simulink model "FinalSim"  (R2022b)
settings: Solver=VariableStepAuto  StartTime=0.0  StopTime=10  RelTol=1e-3
libraries: eeGeneralControl x3
(part 7 of 7)

== system FinalSim/Shoulder Transverse Model/Shoulder Transverse Flexors1/fascicles (CE & PE)/Type F Motor Units/Motor Unit 3 ==
  fenv : Inport
  Y,L : Inport  Port=2
  1/Tf (feff' < 0) : Fcn  Expr=u(2)/(0.02822+0.01513*u(3))
  1/Tf (feff' > 0) : Fcn  Expr=1/(0.02057*u(2)^2+0.0136*u(4))
  1/Ts : Gain  Gain=23.2558  SaturateOnIntegerOverflow=on  OutDataTypeStr=Inherit: Same as input  ParamDataTypeStr=Inherit: Same as input
  Af : Fcn  Expr=1-exp(-(u(1)*u(4)*u(3)/(0.56*u(2)))^u(2))
  Leff' : Fcn  Expr=(u(2)-u(1))^3/((1-u(3))*8.8e-005)
  Leff'->Leff : Integrator  InitialCondition=1
  "Leff,L, Af,fenv" : Mux
  S and old S diff : Sum  Inputs=-+  InputSameDT=on  SaturateOnIntegerOverflow=on  OutDataTypeStr=Inherit: Same as first input
  Y,nf,feff,S : Mux
  aS1 : Constant  Value=1.76
  aS2 : Constant  Value=0.96
  demux Y,L : Demux  Outputs=2
      settings: DisplayOption=none
  feff' : Product  InputSameDT=on  RndMeth=Zero  SaturateOnIntegerOverflow=on  OutDataTypeStr=Inherit: Same as first input
  feff' > 0? : Switch
  feff'->feff : Integrator
  feff>0.1? : Switch  Threshold=0.1
  fenv-fint : Sum  Inputs=+-  InputSameDT=on  SaturateOnIntegerOverflow=on  OutDataTypeStr=Inherit: Same as first input
  fint' : Product  InputSameDT=on  RndMeth=Zero  SaturateOnIntegerOverflow=on  OutDataTypeStr=Inherit: Same as first input
  fint'->fint : Integrator
  fint-feff : Sum  Inputs=+-  InputSameDT=on  SaturateOnIntegerOverflow=on  OutDataTypeStr=Inherit: Same as first input
  nf : Fcn  Expr=2.11+3.31*(1/u-1)
  s'->s : Integrator  InitialCondition=1.76
  A : Outport
  wires:
  Y,L/1 -> demux Y,L/1
  demux Y,L/1 -> Y,nf,feff,S/1
  demux Y,L/2 -> "Leff,L, Af,fenv"/2
  "Leff,L, Af,fenv"/1 -> 1/Tf (feff' < 0)/1, Leff'/1, 1/Tf (feff' > 0)/1
  1/Tf (feff' > 0)/1 -> feff' > 0?/1
  1/Tf (feff' < 0)/1 -> feff' > 0?/3
  fenv/1 -> fenv-fint/1, "Leff,L, Af,fenv"/4
  fenv-fint/1 -> fint'/2
  fint'/1 -> fint'->fint/1
  fint'->fint/1 -> fint-feff/1, fenv-fint/2
  fint-feff/1 -> feff'/2, feff' > 0?/2
  feff' > 0?/1 -> feff'/1, fint'/1
  feff'/1 -> feff'->feff/1
  feff'->feff/1 -> fint-feff/2, Y,nf,feff,S/3, feff>0.1?/2
  Y,nf,feff,S/1 -> Af/1
  Af/1 -> "Leff,L, Af,fenv"/3, A/1
  Leff'/1 -> Leff'->Leff/1
  Leff'->Leff/1 -> "Leff,L, Af,fenv"/1, nf/1
  nf/1 -> Y,nf,feff,S/2
  aS2/1 -> feff>0.1?/1
  aS1/1 -> feff>0.1?/3
  feff>0.1?/1 -> S and old S diff/2
  S and old S diff/1 -> 1/Ts/1
  1/Ts/1 -> s'->s/1
  s'->s/1 -> S and old S diff/1, Y,nf,feff,S/4

== system FinalSim/Shoulder Transverse Model/Shoulder Transverse Flexors1/fascicles (CE & PE)/Type S Motor Units/Motor Unit 1 ==
  fenv : Inport
  Y,L : Inport  Port=2
  1/Tf (feff' < 0) : Fcn  Expr=u(2)/(0.047033+0.025217*u(3))
  1/Tf (feff' > 0) : Fcn  Expr=1/(0.034283*u(2)^2+0.022667*u(4))
  Af : Fcn  Expr=1-exp(-(u(1)*u(4)*u(3)/(0.56*u(2)))^u(2))
  Leff' : Fcn  Expr=(u(2)-u(1))^3/((1-u(3))*8.8e-005)
  Leff'->Leff : Integrator  InitialCondition=1
  "Leff,L, Af,fenv" : Mux
  Y,nf,feff,S : Mux
  aS : Constant
  demux Y,L : Demux  Outputs=2
      settings: DisplayOption=none
  feff' : Product  InputSameDT=on  RndMeth=Zero  SaturateOnIntegerOverflow=on  OutDataTypeStr=Inherit: Same as first input
  feff' > 0? : Switch
  feff'->feff : Integrator
  fenv-fint : Sum  Inputs=+-  InputSameDT=on  SaturateOnIntegerOverflow=on  OutDataTypeStr=Inherit: Same as first input
  fint' : Product  InputSameDT=on  RndMeth=Zero  SaturateOnIntegerOverflow=on  OutDataTypeStr=Inherit: Same as first input
  fint'->fint : Integrator
  fint-feff : Sum  Inputs=+-  InputSameDT=on  SaturateOnIntegerOverflow=on  OutDataTypeStr=Inherit: Same as first input
  nf : Fcn  Expr=2.11+5*(1/u-1)
  A : Outport
  wires:
  Y,L/1 -> demux Y,L/1
  demux Y,L/1 -> Y,nf,feff,S/1
  demux Y,L/2 -> "Leff,L, Af,fenv"/2
  "Leff,L, Af,fenv"/1 -> 1/Tf (feff' < 0)/1, Leff'/1, 1/Tf (feff' > 0)/1
  1/Tf (feff' > 0)/1 -> feff' > 0?/1
  1/Tf (feff' < 0)/1 -> feff' > 0?/3
  fenv/1 -> fenv-fint/1, "Leff,L, Af,fenv"/4
  fenv-fint/1 -> fint'/2
  fint'/1 -> fint'->fint/1
  fint'->fint/1 -> fint-feff/1, fenv-fint/2
  fint-feff/1 -> feff'/2, feff' > 0?/2
  feff' > 0?/1 -> feff'/1, fint'/1
  feff'/1 -> feff'->feff/1
  feff'->feff/1 -> Y,nf,feff,S/3, fint-feff/2
  Y,nf,feff,S/1 -> Af/1
  Af/1 -> "Leff,L, Af,fenv"/3, A/1
  Leff'/1 -> Leff'->Leff/1
  Leff'->Leff/1 -> "Leff,L, Af,fenv"/1, nf/1
  nf/1 -> Y,nf,feff,S/2
  aS/1 -> Y,nf,feff,S/4

== system FinalSim/Shoulder Transverse Model/Shoulder Transverse Flexors1/fascicles (CE & PE)/Type S Motor Units/Motor Unit 2 ==
  fenv : Inport
  Y,L : Inport  Port=2
  1/Tf (feff' < 0) : Fcn  Expr=u(2)/(0.047033+0.025217*u(3))
  1/Tf (feff' > 0) : Fcn  Expr=1/(0.034283*u(2)^2+0.022667*u(4))
  Af : Fcn  Expr=1-exp(-(u(1)*u(4)*u(3)/(0.56*u(2)))^u(2))
  Leff' : Fcn  Expr=(u(2)-u(1))^3/((1-u(3))*8.8e-005)
  Leff'->Leff : Integrator  InitialCondition=1
  "Leff,L, Af,fenv" : Mux
  Y,nf,feff,S : Mux
  aS : Constant
  demux Y,L : Demux  Outputs=2
      settings: DisplayOption=none
  feff' : Product  InputSameDT=on  RndMeth=Zero  SaturateOnIntegerOverflow=on  OutDataTypeStr=Inherit: Same as first input
  feff' > 0? : Switch
  feff'->feff : Integrator
  fenv-fint : Sum  Inputs=+-  InputSameDT=on  SaturateOnIntegerOverflow=on  OutDataTypeStr=Inherit: Same as first input
  fint' : Product  InputSameDT=on  RndMeth=Zero  SaturateOnIntegerOverflow=on  OutDataTypeStr=Inherit: Same as first input
  fint'->fint : Integrator
  fint-feff : Sum  Inputs=+-  InputSameDT=on  SaturateOnIntegerOverflow=on  OutDataTypeStr=Inherit: Same as first input
  nf : Fcn  Expr=2.11+5*(1/u-1)
  A : Outport
  wires:
  Y,L/1 -> demux Y,L/1
  demux Y,L/1 -> Y,nf,feff,S/1
  demux Y,L/2 -> "Leff,L, Af,fenv"/2
  "Leff,L, Af,fenv"/1 -> 1/Tf (feff' < 0)/1, Leff'/1, 1/Tf (feff' > 0)/1
  1/Tf (feff' > 0)/1 -> feff' > 0?/1
  1/Tf (feff' < 0)/1 -> feff' > 0?/3
  fenv/1 -> fenv-fint/1, "Leff,L, Af,fenv"/4
  fenv-fint/1 -> fint'/2
  fint'/1 -> fint'->fint/1
  fint'->fint/1 -> fint-feff/1, fenv-fint/2
  fint-feff/1 -> feff'/2, feff' > 0?/2
  feff' > 0?/1 -> feff'/1, fint'/1
  feff'/1 -> feff'->feff/1
  feff'->feff/1 -> Y,nf,feff,S/3, fint-feff/2
  Y,nf,feff,S/1 -> Af/1
  Af/1 -> "Leff,L, Af,fenv"/3, A/1
  Leff'/1 -> Leff'->Leff/1
  Leff'->Leff/1 -> "Leff,L, Af,fenv"/1, nf/1
  nf/1 -> Y,nf,feff,S/2
  aS/1 -> Y,nf,feff,S/4

== system FinalSim/Tricep Model/Tricep Group/fascicles (CE & PE)/Type F Motor Units/Motor Unit 1 ==
  fenv : Inport
  Y,L : Inport  Port=2
  1/Tf (feff' < 0) : Fcn  Expr=u(2)/(0.02822+0.01513*u(3))
  1/Tf (feff' > 0) : Fcn  Expr=1/(0.02057*u(2)^2+0.0136*u(4))
  1/Ts : Gain  Gain=23.2558  SaturateOnIntegerOverflow=on  OutDataTypeStr=Inherit: Same as input  ParamDataTypeStr=Inherit: Same as input
  Af : Fcn  Expr=1-exp(-(u(1)*u(4)*u(3)/(0.56*u(2)))^u(2))
  Leff' : Fcn  Expr=(u(2)-u(1))^3/((1-u(3))*8.8e-005)
  Leff'->Leff : Integrator  InitialCondition=1
  "Leff,L, Af,fenv" : Mux
  S and old S diff : Sum  Inputs=-+  InputSameDT=on  SaturateOnIntegerOverflow=on  OutDataTypeStr=Inherit: Same as first input
  Y,nf,feff,S : Mux
  aS1 : Constant  Value=1.76
  aS2 : Constant  Value=0.96
  demux Y,L : Demux  Outputs=2
      settings: DisplayOption=none
  feff' : Product  InputSameDT=on  RndMeth=Zero  SaturateOnIntegerOverflow=on  OutDataTypeStr=Inherit: Same as first input
  feff' > 0? : Switch
  feff'->feff : Integrator
  feff>0.1? : Switch  Threshold=0.1
  fenv-fint : Sum  Inputs=+-  InputSameDT=on  SaturateOnIntegerOverflow=on  OutDataTypeStr=Inherit: Same as first input
  fint' : Product  InputSameDT=on  RndMeth=Zero  SaturateOnIntegerOverflow=on  OutDataTypeStr=Inherit: Same as first input
  fint'->fint : Integrator
  fint-feff : Sum  Inputs=+-  InputSameDT=on  SaturateOnIntegerOverflow=on  OutDataTypeStr=Inherit: Same as first input
  nf : Fcn  Expr=2.11+3.31*(1/u-1)
  s'->s : Integrator  InitialCondition=1.76
  A : Outport
  wires:
  Y,L/1 -> demux Y,L/1
  demux Y,L/1 -> Y,nf,feff,S/1
  demux Y,L/2 -> "Leff,L, Af,fenv"/2
  "Leff,L, Af,fenv"/1 -> 1/Tf (feff' < 0)/1, Leff'/1, 1/Tf (feff' > 0)/1
  1/Tf (feff' > 0)/1 -> feff' > 0?/1
  1/Tf (feff' < 0)/1 -> feff' > 0?/3
  fenv/1 -> fenv-fint/1, "Leff,L, Af,fenv"/4
  fenv-fint/1 -> fint'/2
  fint'/1 -> fint'->fint/1
  fint'->fint/1 -> fint-feff/1, fenv-fint/2
  fint-feff/1 -> feff'/2, feff' > 0?/2
  feff' > 0?/1 -> feff'/1, fint'/1
  feff'/1 -> feff'->feff/1
  feff'->feff/1 -> fint-feff/2, Y,nf,feff,S/3, feff>0.1?/2
  Y,nf,feff,S/1 -> Af/1
  Af/1 -> "Leff,L, Af,fenv"/3, A/1
  Leff'/1 -> Leff'->Leff/1
  Leff'->Leff/1 -> "Leff,L, Af,fenv"/1, nf/1
  nf/1 -> Y,nf,feff,S/2
  aS2/1 -> feff>0.1?/1
  aS1/1 -> feff>0.1?/3
  feff>0.1?/1 -> S and old S diff/2
  S and old S diff/1 -> 1/Ts/1
  1/Ts/1 -> s'->s/1
  s'->s/1 -> S and old S diff/1, Y,nf,feff,S/4

== system FinalSim/Tricep Model/Tricep Group/fascicles (CE & PE)/Type F Motor Units/Motor Unit 2 ==
  fenv : Inport
  Y,L : Inport  Port=2
  1/Tf (feff' < 0) : Fcn  Expr=u(2)/(0.02822+0.01513*u(3))
  1/Tf (feff' > 0) : Fcn  Expr=1/(0.02057*u(2)^2+0.0136*u(4))
  1/Ts : Gain  Gain=23.2558  SaturateOnIntegerOverflow=on  OutDataTypeStr=Inherit: Same as input  ParamDataTypeStr=Inherit: Same as input
  Af : Fcn  Expr=1-exp(-(u(1)*u(4)*u(3)/(0.56*u(2)))^u(2))
  Leff' : Fcn  Expr=(u(2)-u(1))^3/((1-u(3))*8.8e-005)
  Leff'->Leff : Integrator  InitialCondition=1
  "Leff,L, Af,fenv" : Mux
  S and old S diff : Sum  Inputs=-+  InputSameDT=on  SaturateOnIntegerOverflow=on  OutDataTypeStr=Inherit: Same as first input
  Y,nf,feff,S : Mux
  aS1 : Constant  Value=1.76
  aS2 : Constant  Value=0.96
  demux Y,L : Demux  Outputs=2
      settings: DisplayOption=none
  feff' : Product  InputSameDT=on  RndMeth=Zero  SaturateOnIntegerOverflow=on  OutDataTypeStr=Inherit: Same as first input
  feff' > 0? : Switch
  feff'->feff : Integrator
  feff>0.1? : Switch  Threshold=0.1
  fenv-fint : Sum  Inputs=+-  InputSameDT=on  SaturateOnIntegerOverflow=on  OutDataTypeStr=Inherit: Same as first input
  fint' : Product  InputSameDT=on  RndMeth=Zero  SaturateOnIntegerOverflow=on  OutDataTypeStr=Inherit: Same as first input
  fint'->fint : Integrator
  fint-feff : Sum  Inputs=+-  InputSameDT=on  SaturateOnIntegerOverflow=on  OutDataTypeStr=Inherit: Same as first input
  nf : Fcn  Expr=2.11+3.31*(1/u-1)
  s'->s : Integrator  InitialCondition=1.76
  A : Outport
  wires:
  Y,L/1 -> demux Y,L/1
  demux Y,L/1 -> Y,nf,feff,S/1
  demux Y,L/2 -> "Leff,L, Af,fenv"/2
  "Leff,L, Af,fenv"/1 -> 1/Tf (feff' < 0)/1, Leff'/1, 1/Tf (feff' > 0)/1
  1/Tf (feff' > 0)/1 -> feff' > 0?/1
  1/Tf (feff' < 0)/1 -> feff' > 0?/3
  fenv/1 -> fenv-fint/1, "Leff,L, Af,fenv"/4
  fenv-fint/1 -> fint'/2
  fint'/1 -> fint'->fint/1
  fint'->fint/1 -> fint-feff/1, fenv-fint/2
  fint-feff/1 -> feff'/2, feff' > 0?/2
  feff' > 0?/1 -> feff'/1, fint'/1
  feff'/1 -> feff'->feff/1
  feff'->feff/1 -> fint-feff/2, Y,nf,feff,S/3, feff>0.1?/2
  Y,nf,feff,S/1 -> Af/1
  Af/1 -> "Leff,L, Af,fenv"/3, A/1
  Leff'/1 -> Leff'->Leff/1
  Leff'->Leff/1 -> "Leff,L, Af,fenv"/1, nf/1
  nf/1 -> Y,nf,feff,S/2
  aS2/1 -> feff>0.1?/1
  aS1/1 -> feff>0.1?/3
  feff>0.1?/1 -> S and old S diff/2
  S and old S diff/1 -> 1/Ts/1
  1/Ts/1 -> s'->s/1
  s'->s/1 -> S and old S diff/1, Y,nf,feff,S/4

== system FinalSim/Tricep Model/Tricep Group/fascicles (CE & PE)/Type F Motor Units/Motor Unit 3 ==
  fenv : Inport
  Y,L : Inport  Port=2
  1/Tf (feff' < 0) : Fcn  Expr=u(2)/(0.02822+0.01513*u(3))
  1/Tf (feff' > 0) : Fcn  Expr=1/(0.02057*u(2)^2+0.0136*u(4))
  1/Ts : Gain  Gain=23.2558  SaturateOnIntegerOverflow=on  OutDataTypeStr=Inherit: Same as input  ParamDataTypeStr=Inherit: Same as input
  Af : Fcn  Expr=1-exp(-(u(1)*u(4)*u(3)/(0.56*u(2)))^u(2))
  Leff' : Fcn  Expr=(u(2)-u(1))^3/((1-u(3))*8.8e-005)
  Leff'->Leff : Integrator  InitialCondition=1
  "Leff,L, Af,fenv" : Mux
  S and old S diff : Sum  Inputs=-+  InputSameDT=on  SaturateOnIntegerOverflow=on  OutDataTypeStr=Inherit: Same as first input
  Y,nf,feff,S : Mux
  aS1 : Constant  Value=1.76
  aS2 : Constant  Value=0.96
  demux Y,L : Demux  Outputs=2
      settings: DisplayOption=none
  feff' : Product  InputSameDT=on  RndMeth=Zero  SaturateOnIntegerOverflow=on  OutDataTypeStr=Inherit: Same as first input
  feff' > 0? : Switch
  feff'->feff : Integrator
  feff>0.1? : Switch  Threshold=0.1
  fenv-fint : Sum  Inputs=+-  InputSameDT=on  SaturateOnIntegerOverflow=on  OutDataTypeStr=Inherit: Same as first input
  fint' : Product  InputSameDT=on  RndMeth=Zero  SaturateOnIntegerOverflow=on  OutDataTypeStr=Inherit: Same as first input
  fint'->fint : Integrator
  fint-feff : Sum  Inputs=+-  InputSameDT=on  SaturateOnIntegerOverflow=on  OutDataTypeStr=Inherit: Same as first input
  nf : Fcn  Expr=2.11+3.31*(1/u-1)
  s'->s : Integrator  InitialCondition=1.76
  A : Outport
  wires:
  Y,L/1 -> demux Y,L/1
  demux Y,L/1 -> Y,nf,feff,S/1
  demux Y,L/2 -> "Leff,L, Af,fenv"/2
  "Leff,L, Af,fenv"/1 -> 1/Tf (feff' < 0)/1, Leff'/1, 1/Tf (feff' > 0)/1
  1/Tf (feff' > 0)/1 -> feff' > 0?/1
  1/Tf (feff' < 0)/1 -> feff' > 0?/3
  fenv/1 -> fenv-fint/1, "Leff,L, Af,fenv"/4
  fenv-fint/1 -> fint'/2
  fint'/1 -> fint'->fint/1
  fint'->fint/1 -> fint-feff/1, fenv-fint/2
  fint-feff/1 -> feff'/2, feff' > 0?/2
  feff' > 0?/1 -> feff'/1, fint'/1
  feff'/1 -> feff'->feff/1
  feff'->feff/1 -> fint-feff/2, Y,nf,feff,S/3, feff>0.1?/2
  Y,nf,feff,S/1 -> Af/1
  Af/1 -> "Leff,L, Af,fenv"/3, A/1
  Leff'/1 -> Leff'->Leff/1
  Leff'->Leff/1 -> "Leff,L, Af,fenv"/1, nf/1
  nf/1 -> Y,nf,feff,S/2
  aS2/1 -> feff>0.1?/1
  aS1/1 -> feff>0.1?/3
  feff>0.1?/1 -> S and old S diff/2
  S and old S diff/1 -> 1/Ts/1
  1/Ts/1 -> s'->s/1
  s'->s/1 -> S and old S diff/1, Y,nf,feff,S/4

== system FinalSim/Tricep Model/Tricep Group/fascicles (CE & PE)/Type S Motor Units/Motor Unit 1 ==
  fenv : Inport
  Y,L : Inport  Port=2
  1/Tf (feff' < 0) : Fcn  Expr=u(2)/(0.047033+0.025217*u(3))
  1/Tf (feff' > 0) : Fcn  Expr=1/(0.034283*u(2)^2+0.022667*u(4))
  Af : Fcn  Expr=1-exp(-(u(1)*u(4)*u(3)/(0.56*u(2)))^u(2))
  Leff' : Fcn  Expr=(u(2)-u(1))^3/((1-u(3))*8.8e-005)
  Leff'->Leff : Integrator  InitialCondition=1
  "Leff,L, Af,fenv" : Mux
  Y,nf,feff,S : Mux
  aS : Constant
  demux Y,L : Demux  Outputs=2
      settings: DisplayOption=none
  feff' : Product  InputSameDT=on  RndMeth=Zero  SaturateOnIntegerOverflow=on  OutDataTypeStr=Inherit: Same as first input
  feff' > 0? : Switch
  feff'->feff : Integrator
  fenv-fint : Sum  Inputs=+-  InputSameDT=on  SaturateOnIntegerOverflow=on  OutDataTypeStr=Inherit: Same as first input
  fint' : Product  InputSameDT=on  RndMeth=Zero  SaturateOnIntegerOverflow=on  OutDataTypeStr=Inherit: Same as first input
  fint'->fint : Integrator
  fint-feff : Sum  Inputs=+-  InputSameDT=on  SaturateOnIntegerOverflow=on  OutDataTypeStr=Inherit: Same as first input
  nf : Fcn  Expr=2.11+5*(1/u-1)
  A : Outport
  wires:
  Y,L/1 -> demux Y,L/1
  demux Y,L/1 -> Y,nf,feff,S/1
  demux Y,L/2 -> "Leff,L, Af,fenv"/2
  "Leff,L, Af,fenv"/1 -> 1/Tf (feff' < 0)/1, Leff'/1, 1/Tf (feff' > 0)/1
  1/Tf (feff' > 0)/1 -> feff' > 0?/1
  1/Tf (feff' < 0)/1 -> feff' > 0?/3
  fenv/1 -> fenv-fint/1, "Leff,L, Af,fenv"/4
  fenv-fint/1 -> fint'/2
  fint'/1 -> fint'->fint/1
  fint'->fint/1 -> fint-feff/1, fenv-fint/2
  fint-feff/1 -> feff'/2, feff' > 0?/2
  feff' > 0?/1 -> feff'/1, fint'/1
  feff'/1 -> feff'->feff/1
  feff'->feff/1 -> Y,nf,feff,S/3, fint-feff/2
  Y,nf,feff,S/1 -> Af/1
  Af/1 -> "Leff,L, Af,fenv"/3, A/1
  Leff'/1 -> Leff'->Leff/1
  Leff'->Leff/1 -> "Leff,L, Af,fenv"/1, nf/1
  nf/1 -> Y,nf,feff,S/2
  aS/1 -> Y,nf,feff,S/4

== system FinalSim/Tricep Model/Tricep Group/fascicles (CE & PE)/Type S Motor Units/Motor Unit 2 ==
  fenv : Inport
  Y,L : Inport  Port=2
  1/Tf (feff' < 0) : Fcn  Expr=u(2)/(0.047033+0.025217*u(3))
  1/Tf (feff' > 0) : Fcn  Expr=1/(0.034283*u(2)^2+0.022667*u(4))
  Af : Fcn  Expr=1-exp(-(u(1)*u(4)*u(3)/(0.56*u(2)))^u(2))
  Leff' : Fcn  Expr=(u(2)-u(1))^3/((1-u(3))*8.8e-005)
  Leff'->Leff : Integrator  InitialCondition=1
  "Leff,L, Af,fenv" : Mux
  Y,nf,feff,S : Mux
  aS : Constant
  demux Y,L : Demux  Outputs=2
      settings: DisplayOption=none
  feff' : Product  InputSameDT=on  RndMeth=Zero  SaturateOnIntegerOverflow=on  OutDataTypeStr=Inherit: Same as first input
  feff' > 0? : Switch
  feff'->feff : Integrator
  fenv-fint : Sum  Inputs=+-  InputSameDT=on  SaturateOnIntegerOverflow=on  OutDataTypeStr=Inherit: Same as first input
  fint' : Product  InputSameDT=on  RndMeth=Zero  SaturateOnIntegerOverflow=on  OutDataTypeStr=Inherit: Same as first input
  fint'->fint : Integrator
  fint-feff : Sum  Inputs=+-  InputSameDT=on  SaturateOnIntegerOverflow=on  OutDataTypeStr=Inherit: Same as first input
  nf : Fcn  Expr=2.11+5*(1/u-1)
  A : Outport
  wires:
  Y,L/1 -> demux Y,L/1
  demux Y,L/1 -> Y,nf,feff,S/1
  demux Y,L/2 -> "Leff,L, Af,fenv"/2
  "Leff,L, Af,fenv"/1 -> 1/Tf (feff' < 0)/1, Leff'/1, 1/Tf (feff' > 0)/1
  1/Tf (feff' > 0)/1 -> feff' > 0?/1
  1/Tf (feff' < 0)/1 -> feff' > 0?/3
  fenv/1 -> fenv-fint/1, "Leff,L, Af,fenv"/4
  fenv-fint/1 -> fint'/2
  fint'/1 -> fint'->fint/1
  fint'->fint/1 -> fint-feff/1, fenv-fint/2
  fint-feff/1 -> feff'/2, feff' > 0?/2
  feff' > 0?/1 -> feff'/1, fint'/1
  feff'/1 -> feff'->feff/1
  feff'->feff/1 -> Y,nf,feff,S/3, fint-feff/2
  Y,nf,feff,S/1 -> Af/1
  Af/1 -> "Leff,L, Af,fenv"/3, A/1
  Leff'/1 -> Leff'->Leff/1
  Leff'->Leff/1 -> "Leff,L, Af,fenv"/1, nf/1
  nf/1 -> Y,nf,feff,S/2
  aS/1 -> Y,nf,feff,S/4

== matlab function FinalSim/Length to Bicep ==
  data: c input; Hb output
function Hb = fcn(c)
% This block supports the Embedded MATLAB subset.
% See the help menu for details. 

a = 0.02919;
b = 0.13581;
s = (a + b + c)/2;

Area = sqrt(s*(s-a)*(s-b)*(s-c));

Hb = 2*Area/c;

== matlab function FinalSim/Length to T. Flexor ==
  data: c input; Hst output
function Hst = fcn(c)
% This block supports the Embedded MATLAB subset.
% See the help menu for details. 

d = 0.08127;
f = 0.014819;
s = (d + f + c)/2;

Area = sqrt(s*(s-d)*(s-f)*(s-c));

Hst = 2*Area/c;

== matlab function FinalSim/ShoulderAbductorPos  ==
  data: u input; y output
function y  = fcn(u)

if u(1,3)<0
    extend = 1;
else
    extend = 0;
end

length = sqrt(u(1,1)^2+u(1,2)^2+u(1,3)^2);

angle = abs(acos((u(1,3))/length));

drive =abs(extend * (length*cos(angle)));
% a = drive;

if drive > 0 
    y = 1/(1+exp(-4*(13*drive-0.43)));
else
    y = 0;
end

== matlab function FinalSim/Length to Bicep3 ==
  data: Sang input; STPos output; APos output
function [STPos, APos] = fcn(Sang)
% This block supports the Embedded MATLAB subset.
% See the help menu for details. 

d = 0.09562;
f = 0.02158;

STPos = sqrt(d^2+f^2-2*d*f*cos(pi-Sang));

e = 0.07125;

APos = sqrt(e^2+f^2-2*e*f*cos(Sang));

== matlab function FinalSim/Length to Adductor ==
  data: c input; Hst output
function Hst = fcn(c)
% This block supports the Embedded MATLAB subset.
% See the help menu for details. 

d = 0.09562;
f = 0.02158;
s = (d + f + c)/2;

Area = sqrt(s*(s-d)*(s-f)*(s-c));

Hst = 2*Area/c;

== matlab function FinalSim/Embedded Vision ==
  data: Sang1 input; Sang2 input; pos output; Eang input
function pos = fcn(Sang1, Sang2, Eang)
% This block supports the Embedded MATLAB subset.
% See the help menu for details. 

UpperArm = 0.175; % Shoulder to elbow
LowerArm = 0.175; % Elbow to wrist

pos = [(UpperArm*cos(Sang2)+LowerArm*cos(Eang+Sang2))*cos(Sang1), (UpperArm*cos(Sang2)+LowerArm*cos(Eang+Sang2))*sin(Sang1), (UpperArm*sin(Sang2)+LowerArm*sin(Eang+Sang2))];

== matlab function FinalSim/ErrorFunction ==
  data: u input; y output; stop output
function [y, stop] = fcn(u)
a = (u);

if sqrt (a(1,1)^2+a(1,2)^2+a(1,3)^2)<=0.004
    stop = 1;
    y=[0,0,0];
else
    y = a;
    stop = 0;
end

== matlab function FinalSim/ElbowTricepPos  ==
  data: u input; y output
function y  = fcn(u)

if u(1,2)>0
    extend = 1;
else
    extend = 0;
end

length = sqrt(u(1,1)^2+u(1,2)^2+u(1,3)^2);

angle = abs(acos((u(1,2))/length));

drive =abs(extend * (length*cos(angle)));
% a = drive;

if drive > 0 
    y = 1/(1+exp(-4*(13*drive-0.43)));
else
    y = 0;
end

== matlab function FinalSim/ElbowBicepPos  ==
  data: u input; y output
function y  = fcn(u)

if u(1,2)<0
    extend = 1;
else
    extend = 0;
end

length = sqrt(u(1,1)^2+u(1,2)^2+u(1,3)^2);

angle = abs(acos((u(1,2))/length));

drive =abs(extend * (length*cos(angle)));
% a = drive;

if drive > 0 
    y = 1/(1+exp(-4*(13*drive-0.43)));
else
    y = 0;
end

== matlab function FinalSim/Length to Bicep1 ==
  data: Sang input; STPos output; APos output
function [STPos, APos] = fcn(Sang)
% This block supports the Embedded MATLAB subset.
% See the help menu for details. 

d = 0.08127;
f = 0.014819;

STPos = sqrt(d^2+f^2-2*d*f*cos(pi-Sang));

e = 0.061219;

APos = sqrt(e^2+f^2-2*e*f*cos(Sang));

== matlab function FinalSim/Length to Bicep2 ==
  data: Eang input; TPos output; BPos output
function [TPos, BPos] = fcn(Eang)
% This block supports the Embedded MATLAB subset.
% See the help menu for details. 

TPos = 0.144 + (pi-Eang)*0.009931;

a = 0.02919; % 0.13248; %
b = 0.13581; %0.03252; %

BPos = sqrt(a^2+b^2-2*a*b*cos(Eang));

== matlab function FinalSim/ShoulderFlexorPos  ==
  data: u input; y output
function y  = fcn(u)

if u(1,1)>0
    extend = 1;
else
    extend = 0;
end

length = sqrt(u(1,1)^2+u(1,2)^2+u(1,3)^2);

angle = abs(acos((u(1,1))/length));

drive =abs(extend * (length*cos(angle)));
% a = drive;

if drive > 0 
    y = 1/(1+exp(-4*(13*drive-0.43)));
else
    y = 0;
end

== matlab function FinalSim/ShoulderExtensorPos  ==
  data: u input; y output
function y  = fcn(u)

if u(1,1)<0
    extend = 1;
else
    extend = 0;
end

length = sqrt(u(1,1)^2+u(1,2)^2+u(1,3)^2);

angle = abs(acos((u(1,1))/length));

drive =abs(extend * (length*cos(angle)));
% a = drive;

if drive > 0 
    y = 1/(1+exp(-4*(13*drive-0.43)));
else
    y = 0;
end

== matlab function FinalSim/Length to Abductor ==
  data: c input; Hsa output
function Hsa = fcn(c)
% This block supports the Embedded MATLAB subset.
% See the help menu for details. 

e = 0.08125;
f = 0.03158;
s = (e + f + c)/2;

Area = sqrt(s*(s-e)*(s-f)*(s-c));

Hsa = 2*Area/c;

== matlab function FinalSim/ShoulderAdductorPos  ==
  data: u input; y output
function y  = fcn(u)

if u(1,3)>0
    extend = 1;
else
    extend = 0;
end

length = sqrt(u(1,1)^2+u(1,2)^2+u(1,3)^2);

angle = abs(acos((u(1,3))/length));

drive =abs(extend * (length*cos(angle)));
% a = drive;

if drive > 0 
    y = 1/(1+exp(-4*(13*drive-0.43)));
else
    y = 0;
end

== matlab function FinalSim/Length to Extensor ==
  data: c input; Hsa output
function Hsa = fcn(c)
% This block supports the Embedded MATLAB subset.
% See the help menu for details. 

e = 0.061219;
f = 0.014819;
s = (e + f + c)/2;

Area = sqrt(s*(s-e)*(s-f)*(s-c));

Hsa = 2*Area/c;
